simulink library "TrajectoryLib"  (R2023a)
settings: Solver=VariableStepAuto  StartTime=0.0  StopTime=10.0  RelTol=1e-3
values from neighbouring files (symbols this model uses):
  eePositions = pchip(tWaypoints,wayPoints',linspace(0,waypointTime,numPoints))    [createWaypoints.m]
  wayPoints = [0.3, 0, 0.630 ... (first row only)    [createWaypoints.m]
undefined symbols (not defined in the file or in its folder): trajectory, wayPointsLoc, X, Y, Z
libraries: sm_lib x15
settings Model: Creator=josea  LastModifiedBy=abirdas
settings SolverCC: AlgebraicLoopSolver=TrustRegion
settings DataIOCC: ReturnWorkspaceOutputs=off
settings DebuggingCC: UnconnectedInputMsg=warning  UnconnectedOutputMsg=warning  UnconnectedLineMsg=warning  ArithmeticOperatorsInVariantConditions=warning
settings ModelReferenceCC: EnableRefExpFcnMdlSchedulingChecks=on
settings SFSimCC: SimUseLocalCustomCode=off  CustomCodeUndefinedFunction=UseInterfaceOnly
settings RTWCC: RTWUseLocalCustomCode=off

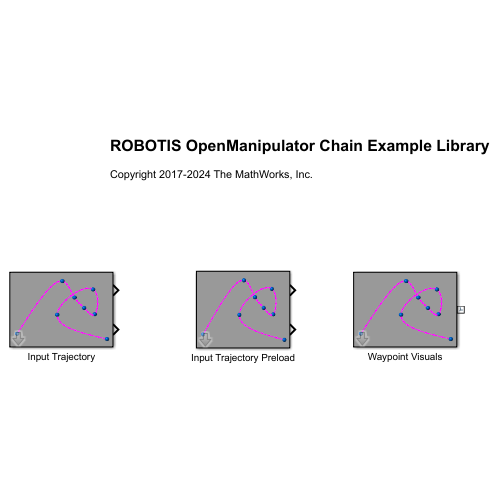
[thumbnail: Simulink's stored preview of the top-level diagram]
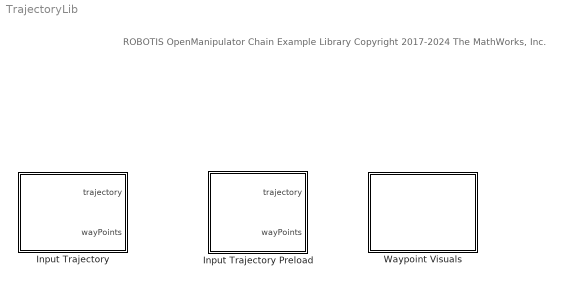
== system TrajectoryLib ==
  note: ROBOTIS OpenManipulator Chain Example Library
      |
      | Copyright 2017-2024 The MathWorks, Inc.
  Input Trajectory : Subsystem  mask(Input Trajectory){numPts=20, scenarioSelection=Stacking 1, trajSelection=Cubic}
      mask prompts: numPts "Number of points"; scenarioSelection "Scenario"; trajSelection "Trajectory type"
      mask help: This subsystem initializes data for the desired trajectory and waypoints. The necessary variables are created in the MATLAB workspace. Two trajectory type options are provided, PCHIP (Piecewise Cubic Hermite Interpolating Polynomial) and Cubic polynomial trajectory.
      mask init:
      | scenario = get_param(gcb,'scenarioSelection');
      | switch scenario
      |     case 'Stacking 1'
      |         scenarioNum = 1;
      |     case 'Stacking 2'
      |         scenarioNum = 2;
      |     case 'Stacking 3'
      |         scenarioNum = 3;
      | end
      | 
      | traj = get_param(gcb,'trajSelection');
      | switch traj
      |     case 'Cubic'
      |         trajNum = 1;
      |     case 'PCHIP'
      |         trajNum = 2;
      | end
      | 
      | evalin('base',['[wayPoints,eePositions] = createWaypoints(' num2str(scenarioNum) ',' num2str(trajNum) ',' num2str(numPts) ');']);
      mask TypeOptions scenarioSelection: Stacking 1 | Stacking 2 | Stacking 3
      mask TypeOptions trajSelection: Cubic | PCHIP
      mask Display: image('WaypointsIcon.PNG')
  Input Trajectory Preload : Subsystem  mask(Input Trajectory preload){scenarioSelection=Custom Trajectory}
      mask prompts: scenarioSelection "Scenario"
      mask help: This subsystem selects a precomputed configuration for trajectory from available scenarios. The necessary variables are selected from MATLAB workspace.
      mask init:
      | scenario = get_param(gcb,'scenarioSelection');
      | switch scenario
      |     case 'Stacking 1'
      |         scenarioNum = '1';
      |     case 'Stacking 2'
      |         scenarioNum = '2';
      |     case 'Custom Trajectory'
      |         scenarioNum = 'Custom';
      | end
      | 
      | load('robotTrajectoryConfig.mat')
      | evalin('base',['wayPointsLoc = Stacking.waypLoc',num2str(scenarioNum,'%01d'),';']);
      | evalin('base',['eePositions = Stacking.eePositionsStacking',num2str(scenarioNum,'%01d'),';']);
      | evalin('base',['trajectory = Stacking.trajectory',num2str(scenarioNum,'%01d'),';']);
      | evalin('base',['wayPoints = Stacking.wayPointsStacking',num2str(scenarioNum,'%01d'),';']);
      mask TypeOptions scenarioSelection: Stacking 1 | Stacking 2 | Custom Trajectory
      mask DialogControl HyperlinkGroup Prompt: Custom trajectory generator app.
      mask DialogControl AppHyperlink Prompt: Open app
      mask DialogControl AppHyperlink Callback: run('CustomTrajectoryGenApp')
      mask Display: image('WaypointsIcon.PNG'); % Use "Edit Image" on toolstrip to change.
  Waypoint Visuals : Subsystem  mask(Waypoint and Trajectory Visualization){spherePoints=wayPoints, sphereRadius=0.01, sphereColor=[0 0.5 1], splinePoints=eePositions', splineColor=[1 0 1]}
      mask prompts: spherePoints "Sphere positions"; sphereRadius "Sphere radius"; sphereColor "Sphere color"; splinePoints "Trajectory points"; splineColor "Trajectory color"
      mask help:
      | This dynamic subsystem places spheres on the desired waypoints and visualizes a pre-computed trajectory as a 3D spline.
      |
      | Sphere positions and Trajectory points are both vectors for which the first 3 columns correspond to the (X, Y, Z) coordinates of the waypoints or trajectory points.
      |
      | NOTE: Make sure the library link for the subsystem is broken when copied from the library. Otherwise the mask initialization will not be able to modify the subsystem contents.
      mask init:
      | % This initialization routine deletes everything within the mask except the
      | % inport and then rebuilds the subsystem with updated information from the
      | % mask parameters
      | 
      | subsystem = gcb;
      | blocks = find_system(subsystem,'LookUnderMasks','all');
      | 
      | % Delete all previous blocks except the inport
      | for idx = 2:length(blocks)-1
      |     delete_block(blocks{idx})
      | end
      | 
      | % Delete all signals
      | while ~isempty(find_system(subsystem,'LookUnderMasks','all','FindAll','on','type','line'))
      |     lines = find_system(subsystem,'LookUnderMasks','all','FindAll','on','type','line');
      |     delete_line(lines(1))
      | end
      | 
      | %%
      | pos1 = [140 100 180 140];
      | pos2 = [140 170 180 210];
      | 
      | set_param(strcat(subsystem,'/W'),'position',[140 60 180 80])
      | 
      | % Add spline to visualize trajectory
      | add_block('sm_lib/Curves and Surfaces/Spline',strcat(subsystem,'/Trajectory Spline'));
      | set_param(strcat(subsystem,'/Trajectory Spline'),'position',pos1,'Orientation','left');
      | set_param(strcat(subsystem,'/Trajectory Spline'),'DataPoints','splinePoints','EndCOnditionType','Natural','GraphicDiffuseColor','splineColor');
      | add_line(subsystem,strcat('W','/RConn1'),strcat('Trajectory Spline','/Lconn1'));
      | 
      | % Add waypoint sphere visuals
      | for idx = 1:size(spherePoints,1)
      |     pos1 = pos1 + [60 0 60 0];
      |     pos2 = pos2 + [60 0 60 0];
      |     
      |     % Add coordinate transform and set parameters
      |     add_block('sm_lib/Frames and Transforms/Rigid Transform',strcat(subsystem,'/Rigid Transform',num2str(idx)));
      |     set_param(strcat(subsystem,'/Rigid Transform',num2str(idx)),'position',pos1,'Orientation','down');
      |     set_param(strcat(subsystem,'/Rigid Transform',num2str(idx)),'TranslationMethod','Cartesian','TranslationCartesianOffset',strcat('[',num2str(spherePoints(idx,1:3)),']'));
      |     add_line(subsystem,strcat('W','/RConn1'),strcat('Rigid Transform',num2str(idx),'/Lconn1'));
      |     
      |     % Add sphere and set parameters
      |     add_block('sm_lib/Body Elements/Spherical Solid',strcat(subsystem,'/Sphere',num2str(idx)))
      |     set_param(strcat(subsystem,'/Sphere',num2str(idx)),'position',pos2,'GraphicDiffuseColor','sphereColor','SphereRadius','sphereRadius')
      |     add_line(subsystem,strcat('Rigid Transform',num2str(idx),'/Rconn1'),strcat('Sphere',num2str(idx),'/RConn1'));
      |    
      | end
      settings: CopyFcn=set_param(gcb,'LinkStatus','breakWithoutHierarchy');
      mask DialogControl ParameterGroupVar Prompt: Sphere Parameters
      mask DialogControl Container3 Prompt: Spline Parameters
      mask Display: image('WaypointsIcon.PNG'); % Use "Edit Image" on toolstrip to change.

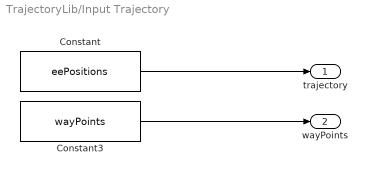
== system TrajectoryLib/Input Trajectory ==
  Constant : Constant  Value=eePositions
  Constant3 : Constant  Value=wayPoints
  trajectory : Outport  VectorParamsAs1DForOutWhenUnconnected=off
  wayPoints : Outport  Port=2  VectorParamsAs1DForOutWhenUnconnected=off
  wires:
  Constant/1 -> trajectory/1
  Constant3/1 -> wayPoints/1

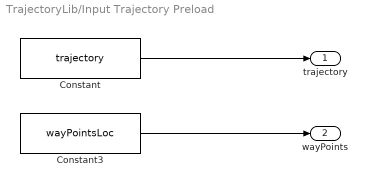
== system TrajectoryLib/Input Trajectory Preload ==
  Constant : Constant  Value=trajectory
  Constant3 : Constant  Value=wayPointsLoc
  trajectory : Outport  VectorParamsAs1DForOutWhenUnconnected=off
  wayPoints : Outport  Port=2  VectorParamsAs1DForOutWhenUnconnected=off
  wires:
  Constant/1 -> trajectory/1
  Constant3/1 -> wayPoints/1

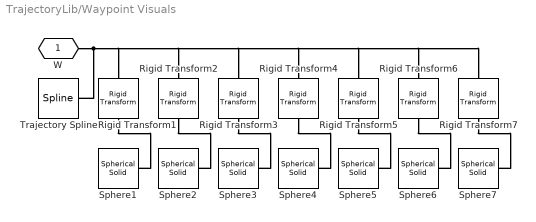
== system TrajectoryLib/Waypoint Visuals ==
  Rigid Transform1 : sm_lib/Frames and Transforms/Rigid Transform  TranslationMethod=Cartesian  TranslationStandardOffset=0  TranslationStandardOffsetUnits=m  TranslationStandardAxis=+Z  TranslationCartesianOffset="[0.3           0        0.63]"  TranslationCartesianOffsetUnits=m  TranslationROffset=0  TranslationROffsetUnits=m  TranslationZOffset=0  TranslationZOffsetUnits=m  TranslationThetaOffset=0  TranslationThetaOffsetUnits=deg  RotationMethod=None  RotationAngleUnits=deg  RotationStandardAxis=+Z  RotationAngle=0.0  RotationArbitraryAxis=[0 0 1]  FollAlignAxisA=+X  BaseAlignAxisA=+Y  FollAlignAxisB=+Y  BaseAlignAxisB=+Z  RotationSequenceAxes=FollowerAxes  RotationSequence=XYX  RotationSequenceAngles=[0 0 0]  RotationSequenceAnglesUnits=deg  RotationMatrix=[1 0 0; 0 1 0; 0 0 1]  Quaternion=[1 0 0 0]
  Rigid Transform2 : sm_lib/Frames and Transforms/Rigid Transform  TranslationMethod=Cartesian  TranslationStandardOffset=0  TranslationStandardOffsetUnits=m  TranslationStandardAxis=+Z  TranslationCartesianOffset="[0.5           0         0.4]"  TranslationCartesianOffsetUnits=m  TranslationROffset=0  TranslationROffsetUnits=m  TranslationZOffset=0  TranslationZOffsetUnits=m  TranslationThetaOffset=0  TranslationThetaOffsetUnits=deg  RotationMethod=None  RotationAngleUnits=deg  RotationStandardAxis=+Z  RotationAngle=0.0  RotationArbitraryAxis=[0 0 1]  FollAlignAxisA=+X  BaseAlignAxisA=+Y  FollAlignAxisB=+Y  BaseAlignAxisB=+Z  RotationSequenceAxes=FollowerAxes  RotationSequence=XYX  RotationSequenceAngles=[0 0 0]  RotationSequenceAnglesUnits=deg  RotationMatrix=[1 0 0; 0 1 0; 0 0 1]  Quaternion=[1 0 0 0]
  Rigid Transform3 : sm_lib/Frames and Transforms/Rigid Transform  TranslationMethod=Cartesian  TranslationStandardOffset=0  TranslationStandardOffsetUnits=m  TranslationStandardAxis=+Z  TranslationCartesianOffset="[0.5           0         0.1]"  TranslationCartesianOffsetUnits=m  TranslationROffset=0  TranslationROffsetUnits=m  TranslationZOffset=0  TranslationZOffsetUnits=m  TranslationThetaOffset=0  TranslationThetaOffsetUnits=deg  RotationMethod=None  RotationAngleUnits=deg  RotationStandardAxis=+Z  RotationAngle=0.0  RotationArbitraryAxis=[0 0 1]  FollAlignAxisA=+X  BaseAlignAxisA=+Y  FollAlignAxisB=+Y  BaseAlignAxisB=+Z  RotationSequenceAxes=FollowerAxes  RotationSequence=XYX  RotationSequenceAngles=[0 0 0]  RotationSequenceAnglesUnits=deg  RotationMatrix=[1 0 0; 0 1 0; 0 0 1]  Quaternion=[1 0 0 0]
  Rigid Transform4 : sm_lib/Frames and Transforms/Rigid Transform  TranslationMethod=Cartesian  TranslationStandardOffset=0  TranslationStandardOffsetUnits=m  TranslationStandardAxis=+Z  TranslationCartesianOffset="[0.5           0         0.2]"  TranslationCartesianOffsetUnits=m  TranslationROffset=0  TranslationROffsetUnits=m  TranslationZOffset=0  TranslationZOffsetUnits=m  TranslationThetaOffset=0  TranslationThetaOffsetUnits=deg  RotationMethod=None  RotationAngleUnits=deg  RotationStandardAxis=+Z  RotationAngle=0.0  RotationArbitraryAxis=[0 0 1]  FollAlignAxisA=+X  BaseAlignAxisA=+Y  FollAlignAxisB=+Y  BaseAlignAxisB=+Z  RotationSequenceAxes=FollowerAxes  RotationSequence=XYX  RotationSequenceAngles=[0 0 0]  RotationSequenceAnglesUnits=deg  RotationMatrix=[1 0 0; 0 1 0; 0 0 1]  Quaternion=[1 0 0 0]
  Rigid Transform5 : sm_lib/Frames and Transforms/Rigid Transform  TranslationMethod=Cartesian  TranslationStandardOffset=0  TranslationStandardOffsetUnits=m  TranslationStandardAxis=+Z  TranslationCartesianOffset="[0.4         0.1         0.2]"  TranslationCartesianOffsetUnits=m  TranslationROffset=0  TranslationROffsetUnits=m  TranslationZOffset=0  TranslationZOffsetUnits=m  TranslationThetaOffset=0  TranslationThetaOffsetUnits=deg  RotationMethod=None  RotationAngleUnits=deg  RotationStandardAxis=+Z  RotationAngle=0.0  RotationArbitraryAxis=[0 0 1]  FollAlignAxisA=+X  BaseAlignAxisA=+Y  FollAlignAxisB=+Y  BaseAlignAxisB=+Z  RotationSequenceAxes=FollowerAxes  RotationSequence=XYX  RotationSequenceAngles=[0 0 0]  RotationSequenceAnglesUnits=deg  RotationMatrix=[1 0 0; 0 1 0; 0 0 1]  Quaternion=[1 0 0 0]
  Rigid Transform6 : sm_lib/Frames and Transforms/Rigid Transform  TranslationMethod=Cartesian  TranslationStandardOffset=0  TranslationStandardOffsetUnits=m  TranslationStandardAxis=+Z  TranslationCartesianOffset="[0.4         0.1        0.16]"  TranslationCartesianOffsetUnits=m  TranslationROffset=0  TranslationROffsetUnits=m  TranslationZOffset=0  TranslationZOffsetUnits=m  TranslationThetaOffset=0  TranslationThetaOffsetUnits=deg  RotationMethod=None  RotationAngleUnits=deg  RotationStandardAxis=+Z  RotationAngle=0.0  RotationArbitraryAxis=[0 0 1]  FollAlignAxisA=+X  BaseAlignAxisA=+Y  FollAlignAxisB=+Y  BaseAlignAxisB=+Z  RotationSequenceAxes=FollowerAxes  RotationSequence=XYX  RotationSequenceAngles=[0 0 0]  RotationSequenceAnglesUnits=deg  RotationMatrix=[1 0 0; 0 1 0; 0 0 1]  Quaternion=[1 0 0 0]
  Rigid Transform7 : sm_lib/Frames and Transforms/Rigid Transform  TranslationMethod=Cartesian  TranslationStandardOffset=0  TranslationStandardOffsetUnits=m  TranslationStandardAxis=+Z  TranslationCartesianOffset="[0.4         0.1         0.4]"  TranslationCartesianOffsetUnits=m  TranslationROffset=0  TranslationROffsetUnits=m  TranslationZOffset=0  TranslationZOffsetUnits=m  TranslationThetaOffset=0  TranslationThetaOffsetUnits=deg  RotationMethod=None  RotationAngleUnits=deg  RotationStandardAxis=+Z  RotationAngle=0.0  RotationArbitraryAxis=[0 0 1]  FollAlignAxisA=+X  BaseAlignAxisA=+Y  FollAlignAxisB=+Y  BaseAlignAxisB=+Z  RotationSequenceAxes=FollowerAxes  RotationSequence=XYX  RotationSequenceAngles=[0 0 0]  RotationSequenceAnglesUnits=deg  RotationMatrix=[1 0 0; 0 1 0; 0 0 1]  Quaternion=[1 0 0 0]
  Sphere{1..7} (7 alike) : sm_lib/Body Elements/Spherical Solid  GraphicAmbientColor=[0.15 0.15 0.15 1.0]  BasedOnType=Density  CenterOfMass=[0 0 0]  CenterOfMassUnits=m  GraphicDiffuseColor=sphereColor  Density=1000  DensityUnits=kg/m^3  DoExposeReferenceFrame=on  GraphicEmissiveColor=[0.0 0.0 0.0 1.0]  ExportEntireGeometry=off  SerializedExposedGeometries=<ExposedGeometries/>  SerializedFrames=<Frames/>  MarkerShape=Sphere  MarkerSize=10  GraphicType=FromGeometry  InertiaType=CalculateFromGeometry  Mass=1  MassUnits=kg  MomentsOfInertia=[1 1 1]  MomentsOfInertiaUnits=kg*m^2  GraphicOpacity=1.0  ProductsOfInertia=[0 0 0]  ProductsOfInertiaUnits=kg*m^2  GraphicShininess=75  GraphicSpecularColor=[0.5 0.5 0.5 1.0]  SphereRadius=sphereRadius  SphereRadiusUnits=m  GraphicVisPropType=SimpleVisualProperties
  Trajectory Spline : sm_lib/Curves and Surfaces/Spline  GraphicAmbientColor=[0.15 0.15 0.15 1.0]  GraphicDiffuseColor=splineColor  DataPoints=splinePoints  DataPointsUnits=m  GraphicEmissiveColor=[0.0 0.0 0.0 1.0]  EndConditionType=Natural  MarkerShape=Sphere  MarkerSize=10  GraphicType=FromGeometry  GraphicOpacity=1.0  GraphicShininess=75  GraphicSpecularColor=[0.5 0.5 0.5 1.0]  GraphicVisPropType=SimpleVisualProperties
  W : PMIOPort  Side=Left
  connections:
  Trajectory Spline/LConn1 -- W/RConn1 -- Rigid Transform1/LConn1 -- Rigid Transform2/LConn1 -- Rigid Transform3/LConn1 -- Rigid Transform4/LConn1 -- Rigid Transform5/LConn1 -- Rigid Transform6/LConn1 -- Rigid Transform7/LConn1
  Rigid Transform1/RConn1 -- Sphere1/RConn1
  Rigid Transform2/RConn1 -- Sphere2/RConn1
  Rigid Transform3/RConn1 -- Sphere3/RConn1
  Rigid Transform4/RConn1 -- Sphere4/RConn1
  Rigid Transform5/RConn1 -- Sphere5/RConn1
  Rigid Transform6/RConn1 -- Sphere6/RConn1
  Rigid Transform7/RConn1 -- Sphere7/RConn1
